simulink model "sat_rise"  (Simulink 7.7)
settings: Solver=ode4  StartTime=0.0  StopTime=35  FixedStep=0.01  RelTol=1e-5
libraries: commchan3 x1
settings Model: Creator=Nic  LastModifiedBy=nic.fischer
settings DebuggingCC: StrictBusMsg=Warning
settings SFSimCC: SimParseCustomCode=off

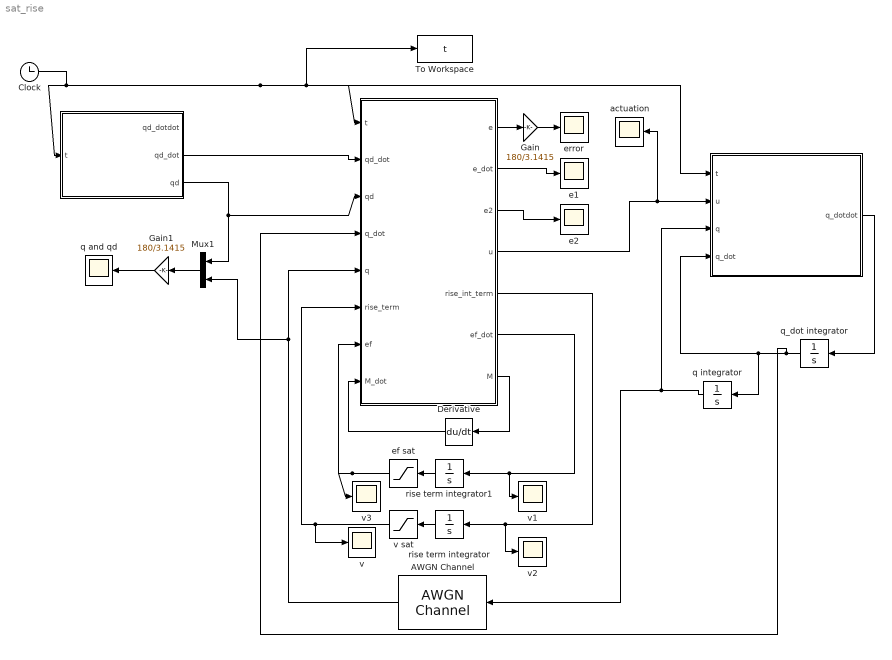
== system sat_rise ==
  "  " : Stateflow chart  TreatAsAtomicUnit=on
  "   " : Stateflow chart  TreatAsAtomicUnit=on
  "    " : Stateflow chart  TreatAsAtomicUnit=on
  AWGN Channel : commchan3/AWGN Channel  SystemSampleTime=-1  InputProcessing=Inherited (this choice will be removed - see release notes)  seed=0  noiseMode="Signal to noise ratio  (SNR)"  EbNodB=10  EsNodB=10  SNRdB=70  bitsPerSym=1  Ps=1  Tsym=1  variance=0.00001
  Clock : Clock
      settings: Decimation=10
  Derivative : Derivative
  Gain : Gain  Gain=180/3.1415
  Gain1 : Gain  Gain=180/3.1415
  Mux1 : Mux  Inputs=2
  To Workspace : ToWorkspace  VariableName=t  SampleTime=-1  SaveFormat=Array
  actuation : Scope
      settings: TimeRange=35  YMin=-300  YMax=300  SaveName=u  DataFormat=Array
  e1 : Scope
      settings: TimeRange=10  YMin=-0.015708814247946  YMax=0.02042832603268958  SaveName=e  DataFormat=Array
  e2 : Scope
      settings: TimeRange=10  YMin=-0.175  YMax=0.2  SaveName=e2  DataFormat=Array
  ef sat : Saturate  UpperLimit=[2;2]  LowerLimit=[-2;-2]
  error : Scope
      settings: TimeRange=35  YMin=-3.343655286613514  YMax=2.486295514732726  SaveName=error  DataFormat=Array
  q and qd : Scope
      settings: TimeRange=35  YMin=-700  YMax=600  SaveName=error1
  q integrator : Integrator  InitialCondition=[100*(pi/180);0]
  q_dot integrator : Integrator  InitialCondition=[0;0]
  rise term integrator : Integrator  InitialCondition=[0;0]
  rise term integrator1 : Integrator  InitialCondition=[0;0]
  v{,1..3} (4 alike) : Scope
      v settings: TimeRange=15  YMin=-3  YMax=3  SaveName=z  DataFormat=Array
      v1 settings: TimeRange=50  YMin=-1.2  YMax=0.5999999999999999  SaveName=ef_dot  DataFormat=Array
      v2 settings: TimeRange=50  YMin=-1.2  YMax=0.5999999999999999  SaveName=v_dot  DataFormat=Array
      v3 settings: TimeRange=40  YMin=-0.275  YMax=0.225  SaveName=z3  DataFormat=Array
  v sat : Saturate  UpperLimit=[3;3]  LowerLimit=[-3;-3]
  wires:
  "   "/1(q_dotdot) -> q_dot integrator/1
  q integrator/1 -> "   "/3(q), AWGN Channel/1
  q_dot integrator/1 -> "   "/4(q_dot), q integrator/1, "  "/4(q_dot)
  Clock/1 -> "   "/1(t), To Workspace/1, "  "/1(t), "    "/1(t)
  "  "/1(e) -> Gain/1
  "    "/3(qd) -> "  "/3(qd), Mux1/1
  Mux1/1 -> Gain1/1
  rise term integrator/1 -> v sat/1
  Gain/1 -> error/1
  Gain1/1 -> q and qd/1
  "    "/2(qd_dot) -> "  "/2(qd_dot)
  v sat/1 -> v/1, "  "/6(rise_term)
  "  "/6(ef_dot) -> rise term integrator1/1, v1/1
  "  "/5(rise_int_term) -> rise term integrator/1, v2/1
  ef sat/1 -> "  "/7(ef), v3/1
  rise term integrator1/1 -> ef sat/1
  "  "/4(u) -> "   "/2(u), actuation/1
  "  "/2(e_dot) -> e1/1
  "  "/3(e2) -> e2/1
  "  "/7(M) -> Derivative/1
  Derivative/1 -> "  "/8(M_dot)
  AWGN Channel/1 -> "  "/5(q), Mux1/2

== matlab function    ==
  data: e output double; e_dot output double; e2 output double; u output double; t input double; qd_dot input double; qd input double; q_dot input double; q input double; rise_term input double; rise_int_term output double; ef input double; ef_dot output double; M output double; M_dot input double
function [e,e_dot,e2,u,rise_int_term,ef_dot,M] = Controller(t,qd_dot,qd,q_dot,q,rise_term,ef,M_dot)

% p1=3.473;
% p2=.193;
% p3=.242;
p1=5.473;
p2=2.193;
p3=1.242;
M  = [ p1+2*p3*cos(q(2))   , p2+p3*cos(q(2));
       p2+p3*cos(q(2))     , p2              ];


%---------------------
% gains
%---------------------
% Rise (full actuation)
% k1 = diag([100,20]);
% beta = diag([10,0.1]);
% alpha1 = diag([40,40]);
% alpha2 = diag([25,25]);

% Rise (reduced gains)
% k1 = diag([40,3]);
% beta = diag([2,2]);
% alpha1 = diag([2,2]);
% alpha2 = diag([1,1]);

% SatRise
%traj 2
% ks = diag([150,15]);
% beta1 = diag([.0001,0.001]);
% beta2 = diag([150,85]);
% alpha1 = diag([2,1.3]);

%traj1 (from parag's dissertation)
gamma1 = diag([30,10]);
gamma2 = diag([20,15]);
beta1 = diag([3,3]);
alpha1 = diag([2,2]);
alpha2 = diag([1,1]);
alpha3 = diag([10,10]);
ks = diag([0.1,0.1]);


%---------------------
% error signals
%---------------------
% rise
e           = qd - q;
e_dot       = qd_dot - q_dot;
% e2          = e_dot + alpha1*e;
e2          = e_dot + alpha1*tanh(e)+tanh(ef);
ef_dot      = ks*diag((cosh(ef)).^2)*(-gamma1*e2 + tanh(e) - gamma2*tanh(ef));

% 

%---------------------
% control design
%---------------------
% % Rise
% rise_int_term = (k1+1)*alpha2*e2+beta*sign(e2);
% u = (k1+1)*e2 + rise_term;

% SatRise
% rise_int_term = beta*diag(cosh(rise_term).^2)*sign(e2);
% u1 = (k1+eye(2))*tanh(e2);
% u2 = k2*tanh(rise_term);
% u = (k1+eye(2))*tanh(e2) + k2*tanh(rise_term);
% for i=1:2
%     if(u(i)>k1(i,i)+k2(i,i)+eye(1)-5) 
%         rise_int_term(i) = 0;
%     elseif(u(i)<-k1(i,i)-k2(i,i)-eye(1)+5)
%         rise_int_term(i) = 0;
%     end
% end

rise_int_term = ks*diag((cosh(rise_term)).^2)*(M*alpha2*tanh(e2) + beta1*sign(e2) + M*alpha3*e2 - alpha1*diag((cosh(e)).^-2)*e2 - M_dot*e2 + gamma2*e2);
u = gamma1*tanh(rise_term);

== matlab function     ==
  data: t input double; q_dotdot output double; u input double; q input double; q_dot input double
function q_dotdot  = Plant(t,u,q,q_dot)

p1=3.473;
p2=.193;
p3=.242;
fd1=5.3;
fd2=1.1;
fs1=8.45;
fs2=2.35;
l1=0.5;
l2=0.5;
M  = [ p1+2*p3*cos(q(2))   , p2+p3*cos(q(2));
       p2+p3*cos(q(2))     , p2              ];
Vm = [ -p3*sin(q(2))*q_dot(2)  , -p3*sin(q(2))*(q_dot(1)+q_dot(2));
        p3*sin(q(2))*q_dot(1)  , 0                                 ];
Fd = diag([fd1,fd2]);
Td = [ 2*sin(t/2) ; 0.2*sin(t/4) ];

%---------------------
% dynamics
%---------------------

% if t>5 && t<6
%     Td=[20*(1-exp(-t^2));0];
% else
%     Td=[0;0];
% end

% T = u - Vm*q_dot - Fd*q_dot;
T = u - Vm*q_dot - Fd*q_dot - Td;
q_dotdot=M\T;

end

== matlab function      ==
  data: qd_dotdot output double; qd_dot output double; t input double; qd output double
function [qd_dotdot,qd_dot,qd] = TrajGen(t)

qd = [(45+60*sin(2*t))*(1-exp(-0.01*t^3))*3.1415/180; -60*(3.1415/180)*sin(2*t)*(1-exp(-0.01*t^3))];
qd_dot = [(6283*t^2*(60*sin(2*t) + 45))/(12000000*exp(t^3/100)) - (6283*cos(2*t)*(1/exp(t^3/100) - 1))/3000;
           (6283*cos(2*t)*(1/exp(t^3/100) - 1))/3000 - (6283*t^2*sin(2*t))/(200000*exp(t^3/100))];
qd_dotdot = [(6283*sin(2*t)*(1/exp(t^3/100) - 1))/1500 + (6283*t^2*cos(2*t))/(50000*exp(t^3/100)) - (18849*t^4*sin(2*t))/(20000000*exp(t^3/100)) + (6283*t*sin(2*t))/(100000*exp(t^3/100));
            (18849*t^4*sin(2*t))/(20000000*exp(t^3/100)) - (6283*t^2*cos(2*t))/(50000*exp(t^3/100)) - (6283*sin(2*t)*(1/exp(t^3/100) - 1))/1500 - (6283*t*sin(2*t))/(100000*exp(t^3/100))];
% qd_dotdot = [-.25*sin(t/2);-4*cos(t)];

% qd = [sin(t);1.5*sin(t)];
% qd_dot = [cos(t);1.5*cos(t)];
end
